simulink model "GMVC_pid2"  (Simulink 5.0)
settings: Solver=ode45  StartTime=0.0  StopTime=500.0  RelTol=1e-3
settings Model: LastModifiedBy=pari

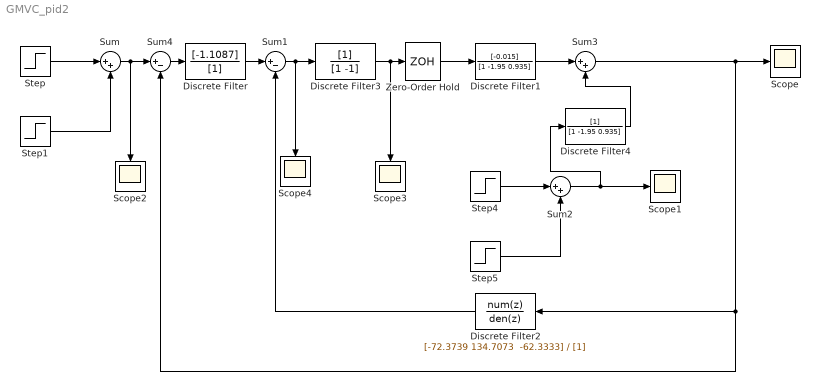
== system GMVC_pid2 ==
  Discrete Filter : DiscreteFilter  Numerator=[-1.1087]  Denominator=[1]
  Discrete Filter1 : DiscreteFilter  Numerator=[-0.015]  Denominator=[1 -1.95 0.935]
  Discrete Filter2 : DiscreteFilter  Orientation=left  Numerator="[-72.3739 134.7073  -62.3333]"  Denominator=[1]
  Discrete Filter3 : DiscreteFilter  Denominator=[1 -1]
  Discrete Filter4 : DiscreteFilter  Denominator=[1 -1.95 0.935]
  Scope{,1..4} (5 alike) : Scope
      Scope settings: TimeRange=1000
      Scope2 settings: Orientation=down  SaveName=ScopeData2
      Scope3 settings: Orientation=down  SaveName=ScopeData3
      Scope4 settings: Orientation=down  SaveName=ScopeData4
  Step : Step  Time=50  SampleTime=1
  Step1 : Step  Time=200  After=-1  SampleTime=1
  Step4 : Step  Time=100  After=0.1  SampleTime=1
  Step5 : Step  Time=150  After=-0.1  SampleTime=1
  Sum : Sum  Inputs=|++  SaturateOnIntegerOverflow=on
  Sum1 : Sum  Inputs=|+-  SaturateOnIntegerOverflow=on
  Sum2 : Sum  Inputs=|++  SaturateOnIntegerOverflow=on
  Sum3 : Sum  Inputs=|++  SaturateOnIntegerOverflow=on
  Sum4 : Sum  Inputs=|+-  SaturateOnIntegerOverflow=on
  Zero-Order Hold : ZeroOrderHold
  wires:
  Step1/1 -> Sum/2
  Step/1 -> Sum/1
  Discrete Filter/1 -> Sum1/1
  Step5/1 -> Sum2/2
  Sum2/1 -> Scope1/1, Discrete Filter4/1
  Discrete Filter1/1 -> Sum3/1
  Sum3/1 -> Scope/1, Discrete Filter2/1, Sum4/2
  Step4/1 -> Sum2/1
  Discrete Filter2/1 -> Sum1/2
  Sum1/1 -> Discrete Filter3/1, Scope4/1
  Discrete Filter3/1 -> Scope3/1, Zero-Order Hold/1
  Zero-Order Hold/1 -> Discrete Filter1/1
  Sum4/1 -> Discrete Filter/1
  Sum/1 -> Sum4/1, Scope2/1
  Discrete Filter4/1 -> Sum3/2
